simulink model "Quad_PID_FUSION_Close_Loop"  (R2023b)
settings: Solver=ode1  StartTime=0.0  StopTime=400  FixedStep=0.01  RelTol=1e-3
values from neighbouring files (symbols this model uses):
  Quad_Model = struct(     'Ixx', 0.016,      'Iyy', 0.016,      'Izz', 0.0274,      'Im', 3.789e-6,      'mass', 1,      'g', 9.8)    [Quad_PID_FUSION_Pipeline.m]    (also in Quad_PID_FUSION_Pipeline_Close_Loop_Attack.m; Quad_PID_FUSION_Pipeline_Close_Loop_Attack_Pipeline.m; Quad_PID_FUSION_Pipeline_Close_Loop_Attack_Pipeline_Reach.m; Quad_PID_FUSION_Pipeline_Close_Loop_Attack_Pipeline_Repeat_V5.m)
  s_x_0 = 0.0    (= 0)    [Quad_PID_FUSION_Pipeline.m]    (also in Quad_PID_FUSION_Pipeline_Loop_Attack_Execution.m = current_norm * cos(angle))
  s_y_0 = 0.0    (= 0)    [Quad_PID_FUSION_Pipeline.m]    (also in Quad_PID_FUSION_Pipeline_Loop_Attack_Execution.m = current_norm * sin(angle))
undefined symbols (not defined in the file or in its folder): DiscIntNeverNeededParam
libraries: simulink x9, rllib x1
(part 2 of 2)

== matlab function Quad_PID_FUSION_Close_Loop/Attack Dynamics ==
  data: X input; s_d output; input input; s input
function s_d = attack_dynamics(X, input,s)


s_d=zeros(12,1);

Quad_Model.Ixx = 0.016;
Quad_Model.Iyy = 0.016;
Quad_Model.Izz = 0.0274;
Quad_Model.Im = 3.789*1e-6;  
Quad_Model.mass = 1;
Quad_Model.g = 9.8;

s_d(1)=s(4);
s_d(2)=s(5);
s_d(3)=s(6);

s_d(4)  =    X(5) *  X(6) * (Quad_Model.Iyy - Quad_Model.Izz) / Quad_Model.Ixx - Quad_Model.Im *  X(5) * 10 + input(1) / Quad_Model.Ixx-...
        ((X(5)-s(5))*  (X(6)-s(6)) * (Quad_Model.Iyy - Quad_Model.Izz) / Quad_Model.Ixx - Quad_Model.Im *  (X(5)-s(5)) * 10 + input(1) / Quad_Model.Ixx);

s_d(5)= X(4) *  X(6) * (Quad_Model.Izz - Quad_Model.Ixx) / Quad_Model.Iyy + Quad_Model.Im *  X(4) * 10 + input(2) / Quad_Model.Iyy-...
        ((X(4)-s(4)) *  (X(6)-s(6)) * (Quad_Model.Izz - Quad_Model.Ixx) / Quad_Model.Iyy + Quad_Model.Im *  (X(4)-s(4)) * 10 + input(2) / Quad_Model.Iyy);

s_d(6)=  X(4) *  X(5) * (Quad_Model.Ixx - Quad_Model.Iyy) / Quad_Model.Izz + input(3) / Quad_Model.Izz-...
        ((X(4)-s(4)) *  (X(5)-s(5)) * (Quad_Model.Ixx - Quad_Model.Iyy) / Quad_Model.Izz + input(3) / Quad_Model.Izz);
        
  
s_d(7)=s(10);
s_d(8)=s(11);
s_d(9)=s(12);


s_d(10) =  (cos(X(1)) * sin(X(2)) * cos(X(3)) + sin(X(1)) * sin(X(3))) * input(4) / Quad_Model.mass - ((cos(X(1)-s(1)) * sin(X(2)-s(2)) * cos(X(3)-s(3)) + sin(X(1)-s(1)) * sin(X(3)-s(3))) * input(4) / Quad_Model.mass);

s_d(11) =  (cos(X(1)) * sin(X(2)) * sin(X(3)) - sin(X(1)) * cos(X(3))) * input(4) / Quad_Model.mass-...
           ((cos(X(1)-s(1)) * sin(X(2)-s(2)) * sin(X(3)-s(3)) - sin(X(1)-s(1)) * cos(X(3)-s(3))) * input(4) / Quad_Model.mass);

s_d(12) =  - Quad_Model.g + cos(X(1)) * cos(X(2)) * input(4) / Quad_Model.mass-(- Quad_Model.g + cos(X(1)-s(1)) * cos(X(2)-s(2)) * input(4) / Quad_Model.mass);

== matlab function Quad_PID_FUSION_Close_Loop/Detector ==
  settings: updateMethod=DISCRETE
  data: x_hat_ekf input; Y input; gamma input; delta_1 input; delta_2 input; r_alarm output; c_alarm output; r output; S_out output
% function [r_alarm, c_alarm, r, S_out] = Detector(x_hat_ekf, Y, gamma, delta_1, delta_2, S_in)
% p = 12;
% n = 12;
% H=eye(12);
% 
% r = norm(Y-H*x_hat_ekf);
% 
% if r > gamma
% 
%     r_alarm = 1;
% 
% else
% 
%     r_alarm = 0;
% 
% end
% 
% 
% S_out = max(0, S_in + r^2 - delta_1);
% 
% 
% if S_out > delta_2
% 
%     c_alarm = 1;
%     % S_out = zeros(12, 12);
% 
% else
% 
%     c_alarm = 0;
% 
% end

function [r_alarm, c_alarm, r, S_out] = Detector(x_hat_ekf, Y, gamma, delta_1, delta_2)
    persistent S;

    % Initialize S only once (ensures it's a scalar)
    if isempty(S)
        S = 0; % Initialize S_in to scalar zero
    end

    % Define system dimensions
    p = 12;
    n = 12;
    H = eye(12);

    % Compute residual norm (scalar)
    r = norm(Y - H * x_hat_ekf);

    % Threshold check
    r_alarm = r > gamma;

    % Update S (ensuring it's scalar)
    S = max(0, S + r^2 - delta_1);

    % Cumulative alarm check
    c_alarm = S > delta_2;
    S_out = S;
    
end

== matlab function Quad_PID_FUSION_Close_Loop/GPS Spoofing Attack Dynamics ==
  data: X input; s_d output; s input; Quad_Model input
function s_d = attack_dynamics(X,s, Quad_Model)

input = zeros(4);
input(1)=0;
input(2)=0;
input(3)=0;
input(4)=0;


s_d=zeros(12,1);

% Quad_Model.Ixx = 0.016;
% Quad_Model.Iyy = 0.016;
% Quad_Model.Izz = 0.0274;
% Quad_Model.Im = 3.789*1e-6;  
% Quad_Model.mass = 1;
% Quad_Model.g = 9.8;

s_d(1)=s(4);
s_d(2)=s(5);
s_d(3)=s(6);

s_d(4)  =    X(5) *  X(6) * (Quad_Model.Iyy - Quad_Model.Izz) / Quad_Model.Ixx - Quad_Model.Im *  X(5) * 10 + input(1) / Quad_Model.Ixx-...
        ((X(5)-s(5))*  (X(6)-s(6)) * (Quad_Model.Iyy - Quad_Model.Izz) / Quad_Model.Ixx - Quad_Model.Im *  (X(5)-s(5)) * 10 + input(1) / Quad_Model.Ixx);

s_d(5)= X(4) *  X(6) * (Quad_Model.Izz - Quad_Model.Ixx) / Quad_Model.Iyy + Quad_Model.Im *  X(4) * 10 + input(2) / Quad_Model.Iyy-...
        ((X(4)-s(4)) *  (X(6)-s(6)) * (Quad_Model.Izz - Quad_Model.Ixx) / Quad_Model.Iyy + Quad_Model.Im *  (X(4)-s(4)) * 10 + input(2) / Quad_Model.Iyy);

s_d(6)=  X(4) *  X(5) * (Quad_Model.Ixx - Quad_Model.Iyy) / Quad_Model.Izz + input(3) / Quad_Model.Izz-...
        ((X(4)-s(4)) *  (X(5)-s(5)) * (Quad_Model.Ixx - Quad_Model.Iyy) / Quad_Model.Izz + input(3) / Quad_Model.Izz);
        
  
% s_d(7)=s(10);
% s_d(8)=s(11);

s_d(7)=s(10);
s_d(8)=s(11);
s_d(9)=s(12);


s_d(10) =  (cos(X(1)) * sin(X(2)) * cos(X(3)) + sin(X(1)) * sin(X(3))) * input(4) / Quad_Model.mass - ((cos(X(1)-s(1)) * sin(X(2)-s(2)) * cos(X(3)-s(3)) + sin(X(1)-s(1)) * sin(X(3)-s(3))) * input(4) / Quad_Model.mass);

s_d(11) =  (cos(X(1)) * sin(X(2)) * sin(X(3)) - sin(X(1)) * cos(X(3))) * input(4) / Quad_Model.mass-...
           ((cos(X(1)-s(1)) * sin(X(2)-s(2)) * sin(X(3)-s(3)) - sin(X(1)-s(1)) * cos(X(3)-s(3))) * input(4) / Quad_Model.mass);

s_d(12) =  - Quad_Model.g + cos(X(1)) * cos(X(2)) * input(4) / Quad_Model.mass-(- Quad_Model.g + cos(X(1)-s(1)) * cos(X(2)-s(2)) * input(4) / Quad_Model.mass);

== matlab function Quad_PID_FUSION_Close_Loop/GPS Sensor ==
  settings: updateMethod=DISCRETE
  data: gps_pos output; input_pos input; input_vel input; gps_position_noise input; gps_velocity_noise input; gps_vel output
function [gps_pos, gps_vel] = Observation(input_pos, input_vel, gps_position_noise, gps_velocity_noise)

gps_pos = input_pos + gps_position_noise;
gps_vel = input_vel + gps_velocity_noise;

== matlab function Quad_PID_FUSION_Close_Loop/Attacker Observation ==
  data: pos input; victim_pos output; vel input; victim_vel output; attacker_noise input
function [victim_pos, victim_vel] = attack_observation(pos, vel, attacker_noise)

victim_pos = zeros(3, 1);
victim_vel = zeros(3, 1);
victim_pos(1) = pos(1) + attacker_noise(1);
victim_pos(2) = pos(2) + attacker_noise(2);
victim_pos(3) = pos(3) + attacker_noise(3);

victim_vel(1) = vel(1) + attacker_noise(4);
victim_vel(2) = vel(2) + attacker_noise(5);
victim_vel(3) = vel(3) + attacker_noise(6);

end

== matlab function Quad_PID_FUSION_Close_Loop/Attacker redirection ==
  settings: updateMethod=DISCRETE
  data: p_control_angle output size=1; p_control_position_x output size=1; p_control_position_y output size=1; theta output size=1; current_theta output size=1; direction_diff output size=1; gamma output size=1; beta output size=1; error_x output size=1; error_y output size=1; new_s_vx output size=1; new_s_vy output size=1; target_pos input; target_radius input; pos input; vel input; s_norm_lim input; delta_s_lim input; dt input; delta_s output size=1
function [p_control_angle, p_control_position_x, p_control_position_y, theta, current_theta, direction_diff, gamma, beta, error_x, error_y, new_s_vx, new_s_vy, delta_s] = ...
    attack_redirection(target_pos, target_radius, pos, vel, s_norm_lim, delta_s_lim, dt)

    % Declare persistent variables for PID errors
    persistent angle_integral_error angle_prev_error pos_integral_error_x pos_prev_error_x pos_integral_error_y pos_prev_error_y prev_s_vx prev_s_vy

    % Initialize persistent variables on first run
    if isempty(angle_integral_error)
        angle_integral_error = 0;
        angle_prev_error = 0;
        pos_integral_error_x = 0;
        pos_prev_error_x = 0;
        pos_integral_error_y = 0;
        pos_prev_error_y = 0;
        prev_s_vx = 0;
        prev_s_vy = 0;
    end

    %% ======= Position and direction errors =======
    % Position error in polar coordinates
    error_x = target_pos(1) - pos(1);
    error_y = target_pos(2) - pos(2);
    r = sqrt(error_x^2 + error_y^2);  % Radial distance to target
    theta = atan2(error_y, error_x);  % Target direction in polar coordinates

    % Velocity in polar coordinates
    v_x = vel(1);
    v_y = vel(2);
    v_mag = sqrt(v_x^2 + v_y^2);  % Velocity magnitude
    current_theta = atan2(v_y, v_x);  % Current velocity direction

    % Compute direction difference (ensuring range [-pi, pi])
    % direction_diff = theta - current_theta;
    direction_diff = mod(theta - current_theta + pi, 2*pi) - pi;
    
    %% ======= PID Controller-Angular =======
    Kp = 1;  % Proportional gain
    Ki = 0.005; % Integral gain
    Kd = 0.001; % Derivative gain

    % Update integral error (accumulated error over time)
    angle_integral_error = angle_integral_error + direction_diff * dt;

    % Compute derivative error (rate of change of error)
    derivative_error = (direction_diff - angle_prev_error) / dt;

    % Compute PID control signal
    % w = min(1, r / 1.0);  % Smoothly reduces for errors < 1m
    % w = 1 - exp(-0.5 * r);

    % Inverted Exponential Decay
    % k = 0.01;  % Adjust decay speed
    % w = 0.1 + (1 - 0.1) * exp(-k * r);
    
    % Sigmoid decay
    r0 = 100; % Midpoint of transition
    k = 0.5; % Steepness of transition
    w = 0.1 + (0.9 ./ (1 + exp(k * (r - r0))));

    Kp_adaptive = Kp * w;
    p_control_angle = Kp_adaptive * direction_diff + Ki * angle_integral_error + Kd * derivative_error;
    p_control_angle = abs(p_control_angle);

    % Update previous error for next iteration
    angle_prev_error = direction_diff;

    % ======= Compute Attack Angle Adjustment (gamma) =======
    gamma = atan(s_norm_lim / (s_norm_lim + v_mag)) * min(1, abs(direction_diff) / pi);

    % Compute beta using atan2 instead of acos
    % beta = atan2(error_y, error_x) + Kp_adaptive*(direction_diff);
    beta = atan2(error_y, error_x) + Kp_adaptive*(direction_diff); % + sign(direction_diff) * gamma;
    % beta = current_theta + p_control_angle*(direction_diff); %+ sign(direction_diff) * gamma;
    beta = mod(beta + pi, 2*pi) - pi;


    %% ======= PID Controller-Position =======
    Kp_pos = 0.1;
    Ki_pos = 0.00;
    Kd_pos = 0.00;

    % Update intergral and derivative errors
    pos_integral_error_x = pos_integral_error_x + error_x * dt;
    pos_derivative_error_x = (error_x - pos_prev_error_x) / dt;

    pos_integral_error_y = pos_integral_error_y + error_y * dt;
    pos_derivative_error_y = (error_y - pos_prev_error_y) / dt;

    % Compute PID control signal
    p_control_position_x = Kp_pos * error_x + Ki_pos * pos_integral_error_x + Kd_pos * pos_derivative_error_x;
    p_control_position_y = Kp_pos * error_y + Ki_pos * pos_integral_error_y + Kd_pos * pos_derivative_error_y;
    % p_control_position = [p_control_position_x, p_control_position_y];

    % Update previous error for next iteration
    pos_prev_error_x = error_x;
    pos_prev_error_y = error_y;


    %% ======= Attack Signal Generation =======
    
    % Compute attack velocity in Cartesian coordinates
    new_s_vx = s_norm_lim * p_control_angle * cos(beta);
    new_s_vy = s_norm_lim * p_control_angle * sin(beta);


    % ======= Compute the Change in Spoofing Velocity (Delta S) =======
    delta_s = sqrt((new_s_vx - prev_s_vx)^2 + (new_s_vy - prev_s_vy)^2);

    % ======= Apply Limit on Delta S if r > target_radius =======
    if r > target_radius && delta_s > delta_s_lim
        % Compute current spoofing velocity magnitude
        s_norm = sqrt(new_s_vx^2 + new_s_vy^2);
    
        if s_norm > 0  % Avoid division by zero
            new_s_vx = new_s_vx * (delta_s_lim / delta_s);
            new_s_vy = new_s_vy * (delta_s_lim / delta_s);
        end
    
        % Update delta_s after scaling
        delta_s = delta_s_lim;
    end


    % Update previous spoofing velocity for next iteration
    prev_s_vx = new_s_vx;
    prev_s_vy = new_s_vy;


end

== matlab function Quad_PID_FUSION_Close_Loop/Attack Injection ==
  data: s output size=1; s input; new_vx input; new_vy input
function s   = attack_injection(s, new_vx, new_vy)
    % Ensure s is a column vector
    s(10) = new_vx;
    s(11) = new_vy;

end

== matlab function Quad_PID_FUSION_Close_Loop/Attacker Redirection MPC ==
  settings: updateMethod=DISCRETE
  data: a_s_opt_x output size=1; a_s_opt_y output size=1; new_s_vx output size=1; new_s_vy output size=1; target_pos input; pos input; vel input; a_s_lim input; dt input
function [a_s_opt_x, a_s_opt_y, new_s_vx, new_s_vy] = ...
    attack_redirection_mpc(target_pos, pos, vel, a_s_lim, dt)

    % Declare persistent variables for previous spoofing velocity
    persistent v_s_x v_s_y prev_v_s_x prev_v_s_y

    % Initialize persistent variables on first run
    if isempty(v_s_x)
        v_s_x = 0;
        v_s_y = 0;
        prev_v_s_x = 0;
        prev_v_s_y = 0;
    end

    % Compute velocity state
    v_x = vel(1);
    v_y = vel(2);

    % ======= New MPC Formulation for Position Control =======
    N = 10;  % Prediction horizon
    Q = diag([1, 1, 0.1, 0.1, 0.1, 0.1]); % Stronger push toward the target
    R = 0.01 * eye(2);  % Penalizes excessive spoofing

    % State transition model including position
    A = [1, 0, dt,  0, dt,  0;
         0, 1,  0, dt,  0, dt;
         0, 0,  1,  0,  1,  0;
         0, 0,  0,  1,  0,  1;
         0, 0,  0,  0,  1,  0;
         0, 0,  0,  0,  0,  1];
    
    B = [0, 0;
         0, 0;
         0, 0;
         0, 0;
         dt,  0;
         0, dt];

    % State vector
    x = [pos(1); pos(2); v_x; v_y; v_s_x; v_s_y];

    % Define reference position (p_target)
    p_target = [target_pos(1); target_pos(2); 0; 0; 0; 0];

    % Define quadratic program
    H = B' * Q * B + R;  % Quadratic cost term
    f = (A * x - p_target)' * Q * B;  % Linear cost term

    % disp('H Matrix:'); disp(H);
    % disp('f Vector:'); disp(f);

    
    % Constraints: Limit spoofing acceleration
    A_con = [eye(2); -eye(2)];
    b_con = [a_s_lim; a_s_lim; -a_s_lim; -a_s_lim];
    
    % Solve the QP problem
    options = optimoptions('quadprog', 'Algorithm', 'active-set', 'Display', 'off');
    initial_guess = [0; 0]; % Start with zero acceleration
    a_s_opt = quadprog(H, f', A_con, b_con, [], [], [], [], initial_guess, options);
    a_s_opt_x = a_s_opt(1);
    a_s_opt_y = a_s_opt(2); 
    
    % Apply acceleration to update spoofing velocity
    new_s_vx = prev_v_s_x + dt * a_s_opt(1);
    new_s_vy = prev_v_s_y + dt * a_s_opt(2);
    
    prev_v_s_x = new_s_vx;
    prev_v_s_y = new_s_vy;


end

== matlab function Quad_PID_FUSION_Close_Loop/Attacker redirection1 ==
  settings: updateMethod=DISCRETE
  data: p_control_angle output size=1; theta output size=1; current_theta output size=1; direction_diff output size=1; gamma output size=1; beta output size=1; error_x output size=1; error_y output size=1; new_s_vx output size=1; new_s_vy output size=1; target_pos input; pos input; vel input; s_norm_lim input; delta_s_lim input; dt input; delta_s output size=1
function [p_control_angle, theta, current_theta, direction_diff, gamma, beta, error_x, error_y, new_s_vx, new_s_vy, delta_s] = ...
    attack_redirection(target_pos, pos, vel, s_norm_lim, delta_s_lim, dt)

    % Declare persistent variables for PID errors
    persistent angle_integral_error angle_prev_error prev_s_vx prev_s_vy

    % Initialize persistent variables on first run
    if isempty(angle_integral_error)
        angle_integral_error = 0;
        angle_prev_error = 0;
        prev_s_vx = 0;
        prev_s_vy = 0;
    end

    % Compute position error in polar coordinates
    error_x = target_pos(1) - pos(1);
    error_y = target_pos(2) - pos(2);
    r = sqrt(error_x^2 + error_y^2);  % Radial distance to target
    theta = atan2(error_y, error_x);  % Target direction in polar coordinates

    % % Return if close to target
    % if r < 1
    %     return;
    % end

    % Compute velocity in polar coordinates
    v_x = vel(1);
    v_y = vel(2);
    v_mag = sqrt(v_x^2 + v_y^2);  % Velocity magnitude
    current_theta = atan2(v_y, v_x);  % Current velocity direction

    % Compute direction difference (ensuring range [-pi, pi])
    direction_diff = mod(theta - current_theta + pi, 2*pi) - pi;
    
    % ======= PID Controller =======
    Kp = 0.05;  % Proportional gain
    Ki = 0.005; % Integral gain
    Kd = 0.0001; % Derivative gain

    % Update integral error (accumulated error over time)
    angle_integral_error = angle_integral_error + direction_diff * dt;

    % Compute derivative error (rate of change of error)
    derivative_error = (direction_diff - angle_prev_error) / dt;

    % Compute PID control signal
    % w = min(1, r / 1.0);  % Smoothly reduces for errors < 1m
    w = 1 - exp(-0.02 * r);
    Kp_adaptive = Kp * w;
    p_control_angle = Kp_adaptive * direction_diff + Ki * angle_integral_error + Kd * derivative_error;
    % p_control_angle = abs(p_control_angle);

    % Update previous error for next iteration
    angle_prev_error = direction_diff;

    % ======= Compute Attack Angle Adjustment (gamma) =======
    gamma = atan(s_norm_lim / (s_norm_lim + v_mag)) * min(1, abs(direction_diff) / pi);

    % Compute beta using atan2 instead of acos
    % beta = atan2(error_y, error_x) + sign(direction_diff) * gamma;
    beta = atan2(error_y, error_x) + Kp_adaptive*(direction_diff); %+ sign(direction_diff) * gamma;
    % beta = current_theta + p_control_angle*(direction_diff); %+ sign(direction_diff) * gamma;
    beta = mod(beta + pi, 2*pi) - pi;

    % Compute attack velocity in Cartesian coordinates
    new_s_vx = s_norm_lim * cos(beta);
    new_s_vy = s_norm_lim * sin(beta);

    % Scale spoofing velocity using PID control
    new_s_vx = p_control_angle * new_s_vx;
    new_s_vy = p_control_angle * new_s_vy;

    % ======= Compute the Change in Spoofing Velocity (Delta S) =======
    delta_s = sqrt((new_s_vx - prev_s_vx)^2 + (new_s_vy - prev_s_vy)^2);

    % ======= Apply Limit on Delta S if r > 5m =======
    if r > 5 && delta_s > delta_s_lim
        % Compute current spoofing velocity magnitude
        s_norm = sqrt(new_s_vx^2 + new_s_vy^2);
    
        if s_norm > 0  % Avoid division by zero
            % Compute new scaled spoofing velocity magnitude
            s_norm_scaled = s_norm * (delta_s_lim / delta_s);
    
            % Keep the same attack direction beta, recompute scaled components
            new_s_vx = s_norm_scaled * cos(beta);
            new_s_vy = s_norm_scaled * sin(beta);
        end
    
        % Update delta_s after scaling
        delta_s = delta_s_lim;
    end

    % Update previous spoofing velocity for next iteration
    prev_s_vx = new_s_vx;
    prev_s_vy = new_s_vy;


end

== matlab function Quad_PID_FUSION_Close_Loop/MATLAB Function ==
  data: pos_x input; pos_y input; vel_x input; vel_y input; target input; reward output
function reward = rewardFunction(pos_x, pos_y, vel_x, vel_y, target)

    target_px = target(1);  % Assuming target at (0,0)
    target_py = target(2);

    % Compute position error
    pos_error = sqrt((pos_x - target_px)^2 + (pos_y - target_py)^2);

    % Compute velocity alignment error
    theta = atan2(pos_y - target_py, pos_x - target_px);
    current_theta = atan2(vel_y, vel_x);
    direction_error = abs(theta - current_theta);

    % Reward: Penalize position and direction errors
    reward = -1 * pos_error - 0.1 * direction_error;
end

== matlab function Quad_PID_FUSION_Close_Loop/MATLAB Function1 ==
  data: pos_x input; pos_y input; target input; is_done output
function is_done = isDone(pos_x, pos_y, target)

    target_px = target(1);  % Assuming target at (0,0)
    target_py = target(2);

    % Compute position error
    pos_error = sqrt((pos_x - target_px)^2 + (pos_y - target_py)^2);

    if pos_error < 3
        is_done = true;
    else
        is_done = false;
    end
end

== matlab function Quad_PID_FUSION_Close_Loop/MATLAB Function2 ==
  data: attacker_pos input; attacker_vel input; obs output
function obs = obsFunction(attacker_pos, attacker_vel)

    obs = zeros(4, 1);
    obs(1) = attacker_pos(1);
    obs(2) = attacker_pos(2);
    obs(3) = attacker_vel(1);
    obs(4) = attacker_vel(2);
end

== matlab function Quad_PID_FUSION_Close_Loop/Attacker redirection2 ==
  settings: updateMethod=DISCRETE
  data: p_control_angle output size=1; p_control_position_x output size=1; p_control_position_y output size=1; theta output size=1; current_theta output size=1; direction_diff output size=1; gamma output size=1; beta output size=1; error_x output size=1; error_y output size=1; new_s_vx output size=1; new_s_vy output size=1; target_pos input; target_radius input; pos input; vel input; s_norm_lim input; delta_s_lim input; dt input; delta_s output size=1
function [p_control_angle, p_control_position_x, p_control_position_y, theta, current_theta, direction_diff, gamma, beta, error_x, error_y, new_s_vx, new_s_vy, delta_s] = ...
    attack_redirection(target_pos, target_radius, pos, vel, s_norm_lim, delta_s_lim, dt)

    % Declare persistent variables for PID errors
    persistent angle_integral_error angle_prev_error pos_integral_error_x pos_prev_error_x pos_integral_error_y pos_prev_error_y prev_s_vx prev_s_vy

    % Initialize persistent variables on first run
    if isempty(angle_integral_error)
        angle_integral_error = 0;
        angle_prev_error = 0;
        pos_integral_error_x = 0;
        pos_prev_error_x = 0;
        pos_integral_error_y = 0;
        pos_prev_error_y = 0;
        prev_s_vx = 0;
        prev_s_vy = 0;
    end

    %% ======= Position and direction errors =======
    % Position error in polar coordinates
    error_x = target_pos(1) - pos(1);
    error_y = target_pos(2) - pos(2);
    r = sqrt(error_x^2 + error_y^2);  % Radial distance to target
    theta = atan2(error_y, error_x);  % Target direction in polar coordinates

    % Velocity in polar coordinates
    v_x = vel(1);
    v_y = vel(2);
    v_mag = sqrt(v_x^2 + v_y^2);  % Velocity magnitude
    current_theta = atan2(v_y, v_x);  % Current velocity direction

    % Compute direction difference (ensuring range [-pi, pi])
    % direction_diff = theta - current_theta;
    direction_diff = mod(theta - current_theta + pi, 2*pi) - pi;
    
    %% ======= PID Controller-Angular =======
    Kp = 1;  % Proportional gain
    Ki = 0.005; % Integral gain
    Kd = 0.001; % Derivative gain

    % Update integral error (accumulated error over time)
    angle_integral_error = angle_integral_error + direction_diff * dt;

    % Compute derivative error (rate of change of error)
    derivative_error = (direction_diff - angle_prev_error) / dt;

    % Compute PID control signal
    % w = min(1, r / 1.0);  % Smoothly reduces for errors < 1m
    % w = 1 - exp(-0.5 * r);

    % Inverted Exponential Decay
    % k = 0.01;  % Adjust decay speed
    % w = 0.1 + (1 - 0.1) * exp(-k * r);
    
    % Sigmoid decay
    r0 = 100; % Midpoint of transition
    k = 0.5; % Steepness of transition
    w = 0.1 + (0.9 ./ (1 + exp(k * (r - r0))));

    Kp_adaptive = Kp * w;
    p_control_angle = Kp_adaptive * direction_diff + Ki * angle_integral_error + Kd * derivative_error;
    p_control_angle = abs(p_control_angle);

    % Update previous error for next iteration
    angle_prev_error = direction_diff;

    % ======= Compute Attack Angle Adjustment (gamma) =======
    gamma = atan(s_norm_lim / (s_norm_lim + v_mag)) * min(1, abs(direction_diff) / pi);

    % Compute beta using atan2 instead of acos
    % beta = atan2(error_y, error_x) + Kp_adaptive*(direction_diff);
    beta = atan2(error_y, error_x) + Kp_adaptive*(direction_diff); % + sign(direction_diff) * gamma;
    % beta = current_theta + p_control_angle*(direction_diff); %+ sign(direction_diff) * gamma;
    beta = mod(beta + pi, 2*pi) - pi;


    %% ======= PID Controller-Position =======
    Kp_pos = 0.1;
    Ki_pos = 0.00;
    Kd_pos = 0.00;

    % Update intergral and derivative errors
    pos_integral_error_x = pos_integral_error_x + error_x * dt;
    pos_derivative_error_x = (error_x - pos_prev_error_x) / dt;

    pos_integral_error_y = pos_integral_error_y + error_y * dt;
    pos_derivative_error_y = (error_y - pos_prev_error_y) / dt;

    % Compute PID control signal
    p_control_position_x = Kp_pos * error_x + Ki_pos * pos_integral_error_x + Kd_pos * pos_derivative_error_x;
    p_control_position_y = Kp_pos * error_y + Ki_pos * pos_integral_error_y + Kd_pos * pos_derivative_error_y;
    % p_control_position = [p_control_position_x, p_control_position_y];

    % Update previous error for next iteration
    pos_prev_error_x = error_x;
    pos_prev_error_y = error_y;


    %% ======= Attack Signal Generation =======
    
    % Compute attack velocity in Cartesian coordinates
    new_s_vx = s_norm_lim * p_control_angle * cos(beta);
    new_s_vy = s_norm_lim * p_control_angle * sin(beta);


    % % Update using position control
    % new_s_vx = s_norm_lim * p_control_position_x - v_x;
    % new_s_vy = s_norm_lim * p_control_position_y - v_y;

    % ======= Compute the Change in Spoofing Velocity (Delta S) =======
    delta_s = sqrt((new_s_vx - prev_s_vx)^2 + (new_s_vy - prev_s_vy)^2);

    % ======= Apply Limit on Delta S if r > target_radius =======
    if r > target_radius && delta_s > delta_s_lim
        % Compute current spoofing velocity magnitude
        s_norm = sqrt(new_s_vx^2 + new_s_vy^2);
    
        if s_norm > 0  % Avoid division by zero
            new_s_vx = new_s_vx * (delta_s_lim / delta_s);
            new_s_vy = new_s_vy * (delta_s_lim / delta_s);
        end
    
        % Update delta_s after scaling
        delta_s = delta_s_lim;
    end


    % Update previous spoofing velocity for next iteration
    prev_s_vx = new_s_vx;
    prev_s_vy = new_s_vy;


end

== matlab function Quad_PID_FUSION_Close_Loop/Attacker redirection3 ==
  settings: updateMethod=DISCRETE
  data: current_time input; attack_start_time input; s_vx output size=1; s_vy output size=1; a_sx output size=1; a_sy output size=1; target_pos input; pos input; vel input; dt input; delta_s_lim input; v_ref_x output size=1; v_ref_y output size=1; delta_s_pid output size=1
function [s_vx, s_vy, a_sx, a_sy, v_ref_x, v_ref_y, delta_s_pid] = attack_redirection_cascade_pid(current_time, attack_start_time, target_pos, pos, vel, dt, delta_s_lim)
    % ======= Declare Persistent Variables =======
    persistent integral_pos_x integral_pos_y integral_vel_x integral_vel_y
    persistent prev_error_pos_x prev_error_pos_y prev_error_vel_x prev_error_vel_y
    persistent s_vx_prev s_vy_prev

    % Initialize persistent variables on first run
    if isempty(integral_pos_x)
        integral_pos_x = 0; integral_pos_y = 0;
        integral_vel_x = 0; integral_vel_y = 0;
        prev_error_pos_x = 0; prev_error_pos_y = 0;
        prev_error_vel_x = 0; prev_error_vel_y = 0;
        s_vx_prev = 0; s_vy_prev = 0;  % Initial spoofing velocity
    end

    if current_time >= attack_start_time
    
        % Compute position error
        error_pos_x = target_pos(1) - pos(1);
        error_pos_y = target_pos(2) - pos(2);
        r = sqrt(error_pos_x^2 + error_pos_y^2);
    
        % ======= Outer Loop: Position Control (Computes Desired Velocity) =======
        base_Kp_pos = 0.5;  
        Kp_pos = base_Kp_pos * (1 - exp(-0.1 * r)); 
        % Kp_pos = 0.5;  % Position control proportional gain
        Ki_pos = 0.005; % Position control integral gain
        Kd_pos = 0.1;  % Position control derivative gain
    
        % Prevent integral windup: Reset integral term when error changes sign
        if sign(error_pos_x) ~= sign(prev_error_pos_x)
            integral_pos_x = 0;
        end
        if sign(error_pos_y) ~= sign(prev_error_pos_y)
            integral_pos_y = 0;
        end
    
        % Update integral error for position
        integral_pos_x = integral_pos_x + error_pos_x * dt;
        integral_pos_y = integral_pos_y + error_pos_y * dt;
    
        % Compute derivative error for position
        derivative_error_pos_x = (error_pos_x - prev_error_pos_x) / dt;
        derivative_error_pos_y = (error_pos_y - prev_error_pos_y) / dt;
    
        % Compute desired velocity
        v_x_desired = Kp_pos * error_pos_x + Ki_pos * integral_pos_x + Kd_pos * derivative_error_pos_x;
        v_y_desired = Kp_pos * error_pos_y + Ki_pos * integral_pos_y + Kd_pos * derivative_error_pos_y;
    
        % Apply velocity constraint ||v_desired|| ≤ 5 m/s
        v_desired_norm = sqrt(v_x_desired^2 + v_y_desired^2);
        v_max_limit = 5;  % Maximum desired velocity
        if v_desired_norm > v_max_limit
            v_x_desired = (v_x_desired / v_desired_norm) * v_max_limit;
            v_y_desired = (v_y_desired / v_desired_norm) * v_max_limit;
        end
    
        v_ref_x = v_x_desired;
        v_ref_y = v_y_desired;
    
        % Update previous position error
        prev_error_pos_x = error_pos_x;
        prev_error_pos_y = error_pos_y;
    
        % ======= Inner Loop: Velocity Control (Computes Spoofing Acceleration) =======
        Kp_vel = 0.05;  % Velocity control proportional gain
        Ki_vel = 0.002; % Velocity control integral gain
        Kd_vel = 0.001;  % Velocity control derivative gain
    
        % Compute velocity error
        error_vel_x = v_x_desired - vel(1);
        error_vel_y = v_y_desired - vel(2);
    
        % === Anti-Windup for Velocity Integral ===
        if sign(error_vel_x) ~= sign(prev_error_vel_x)
            integral_vel_x = 0;
        end
        if sign(error_vel_y) ~= sign(prev_error_vel_y)
            integral_vel_y = 0;
        end
    
        % Update integral error for velocity
        integral_vel_x = integral_vel_x + error_vel_x * dt;
        integral_vel_y = integral_vel_y + error_vel_y * dt;
    
        % Compute derivative error for velocity
        derivative_error_vel_x = (error_vel_x - prev_error_vel_x) / dt;
        derivative_error_vel_y = (error_vel_y - prev_error_vel_y) / dt;
    
        % Compute spoofing acceleration
        a_sx = Kp_vel * error_vel_x + Ki_vel * integral_vel_x + Kd_vel * derivative_error_vel_x;
        a_sy = Kp_vel * error_vel_y + Ki_vel * integral_vel_y + Kd_vel * derivative_error_vel_y;
    
        % Apply acceleration constraint ||a_s|| ≤ delta_s_lim
        a_s_norm = sqrt(a_sx^2 + a_sy^2);
        if a_s_norm > delta_s_lim
            a_sx = (a_sx / a_s_norm) * delta_s_lim;
            a_sy = (a_sy / a_s_norm) * delta_s_lim;
        end
    
        delta_s_pid = sqrt(a_sx^2 + a_sy^2);
    
        % Update previous velocity error
        prev_error_vel_x = error_vel_x;
        prev_error_vel_y = error_vel_y;
    
        % ======= Compute Spoofing Velocity =======
        s_vx = s_vx_prev + a_sx * dt;
        s_vy = s_vy_prev + a_sy * dt;
    
        % Update previous spoofing velocity for next iteration
        s_vx_prev = s_vx;
        s_vy_prev = s_vy;
    else
        s_vx = 0;
        s_vy = 0;
        a_sx = 0;  
        a_sy = 0;
        v_ref_x = 0;
        v_ref_y = 0; 
        delta_s_pid = 0;

    end
end

== matlab function Quad_PID_FUSION_Close_Loop/Thrust_to_Attitude ==
  data: thrust_enu_x input; roll_sp output; thrust_enu_y input; thrust_enu_z input; pitch_sp output; yaw_sp output; yaw_setpoint input; thrust_body output
function [roll_sp,pitch_sp, yaw_sp,thrust_body] = Thrust_to_Attitude(thrust_enu_x,thrust_enu_y,thrust_enu_z,yaw_setpoint)

    thrust_sp = [thrust_enu_x;thrust_enu_y;thrust_enu_z];

    yaw_sp = yaw_setpoint;
    
    thrust_sp_length = norm(thrust_sp);
    
    thrust_body = thrust_sp_length;

    if thrust_sp_length > 0.00001 
        body_z = thrust_sp/thrust_sp_length;
    else 
        body_z = [0;0;1];
    end
    
     y_C= [-sin(yaw_sp);cos(yaw_sp);0];

    if abs(body_z(3)) > 0.000001
        body_x = cross( y_C,body_z);
        if body_z(3) < 0.0 
           body_x = -body_x;
        end
        body_x = body_x/norm(body_x);
    else 
        body_x = [0;0;1];
    end
    
    body_y = cross( body_z,body_x);
    
    R_sp = [body_x,body_y,body_z];
    
    euler_sp = rotation_to_euler(R_sp);
    
    roll_sp  = euler_sp(1);
    pitch_sp = euler_sp(2);
    yaw_sp   = euler_sp(3);
end

function euler_angle = rotation_to_euler(dcm)

    euler_angle = zeros(3,1);
    phi_val = atan2(dcm(3, 2), dcm(3, 3));
    theta_val = asin(-dcm(3, 1));
    psi_val = atan2(dcm(2, 1), dcm(1, 1));

    if abs(theta_val - pi / 2.0) < 1.0e-3 
        phi_val = 0.0;
        psi_val = atan2(dcm(2, 3), dcm(1, 3));
    elseif abs(theta_val + pi / 2.0) <  1.0e-3
        phi_val = 0.0;
        psi_val = atan2(-dcm(2, 3), -dcm(1, 3));
    end

    euler_angle(1) = phi_val;
    euler_angle(2) = theta_val;
    euler_angle(3) = psi_val;

end

== matlab function Quad_PID_FUSION_Close_Loop/Position Controller/MATLAB Function ==
  data: thrust_x input; thrust_sp_x output; thrust_y input; thrust_z input; thrust_sp_y output; thtust_sp_z output
function [thrust_sp_x,thrust_sp_y,thtust_sp_z] = Thrust_Limit(thrust_x,thrust_y,thrust_z)

MPC_THR_MIN = 0.1;
MPC_THR_MAX = 0.9;
tilt_max = 20;

thtust_sp_z = constrain_function2( thrust_z, MPC_THR_MIN, MPC_THR_MAX);

thrust_max_XY_tilt = abs(thtust_sp_z) * tan(tilt_max/180.0*pi);
thrust_max_XY = sqrt(MPC_THR_MAX * MPC_THR_MAX - thtust_sp_z * thtust_sp_z);

thrust_max_XY = min(thrust_max_XY_tilt, thrust_max_XY);


if (thrust_x^2 + thrust_y^2) > thrust_max_XY^2 
    mag = sqrt(thrust_x^2 + thrust_y^2);
    thrust_sp_x = thrust_x / mag * thrust_max_XY;
    thrust_sp_y = thrust_y / mag * thrust_max_XY;
else
    thrust_sp_x = thrust_x;
    thrust_sp_y = thrust_y;
end

end
function output = constrain_function2(data, Min, Max)
    
    if data > Max
        output =  Max;
    elseif data < Min
        output = Min;
    else
        output = data;
    end
end
